simulink model "Con_ref_de_vel"  (R2023b)
settings: Solver=VariableStepAuto  StartTime=0.0  StopTime=14  MaxStep=1e-3  RelTol=1e-3
undefined symbols (not defined in the file or in its folder): alpha_Cu, b_a, b_eq, C_ts, g, J_eq, k_l, K_omega, K_sa, K_sia, K_theta, L_d, L_ls, L_q, lambda_m, magnitude, P_p, r, R_0, R_d, R_q, R_sREF, R_tsamb, T_amb, T_sREF
libraries: simulink x12
(part 1 of 2)
settings Model: Creator=MSI  LastModifiedBy=MSI

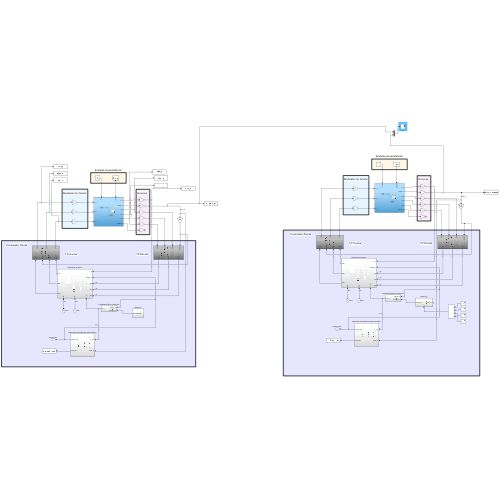
[thumbnail: Simulink's stored preview of the top-level diagram]
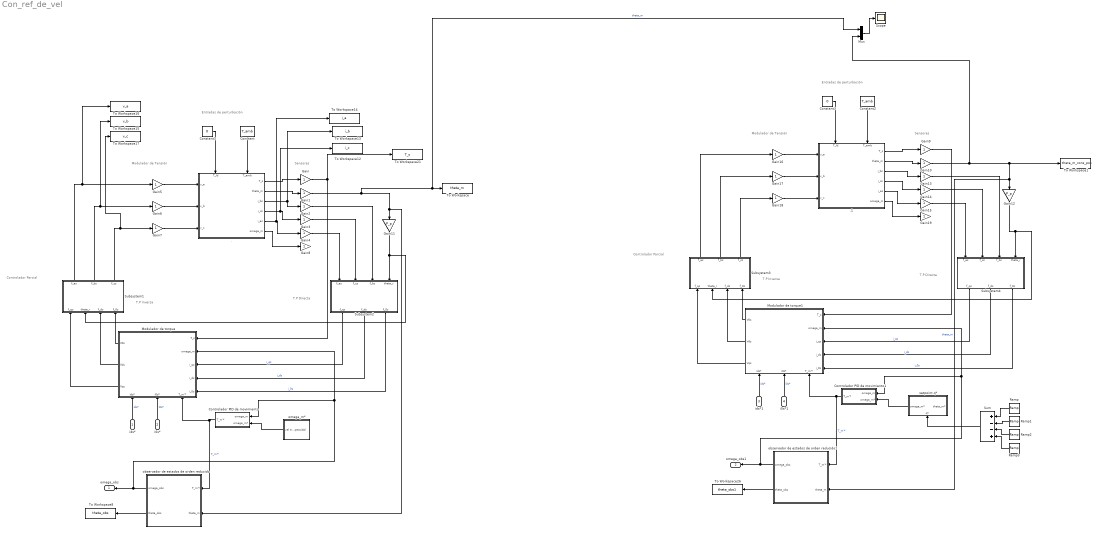
== system Con_ref_de_vel ==
  note: Sensores
  note: T.P Inversa
  note: Entradas de perturbación
  note: Controlador Parcial
  note: T.P Directa
  note: Modulador de Tensión
  note: T.P Directa
  note: Controlador Parcial
  note: Modulador de Tensión
  note: T.P Inversa
  note: Sensores
  note: Entradas de perturbación
  ids* : Inport
  i0s* : Inport  Port=2
  ids*1 : Inport  Port=3
  i0s*1 : Inport  Port=4
  . : Subsystem
      settings: PortSchema="{\"entries\":[{\"content\":{\"sides\":[{\"content\":{\"connectorIds\":[\"In1\",\"In2\",\"In3\"]},\"type\":\"ConnectorPlacement.EquallySpacedRectSide\",\"uuid\":\"a2221977-a2db-4f9f-a6b6-e4e93ab83132\"},{\"content\":{\"connectorIds\":[\"Out1\",\"Out2\",\"Out3\",\"Out4\",\"Out5\",\"Out6\"],\"side\":\"RIGHT\"},\"type\":\"ConnectorPlacement.EquallySpacedRectSide\",\"uuid\":\"4d1b64fb-cd5f-444c-9c55-dd968f667727\"},{\"content\":{\"connectorIds\":[\"In4\",\"In5\"],\"side\":\"TOP\"},\"type\":\"ConnectorPlacement.EquallySpacedRectSide\",\"uuid\":\"feec2d7e-2013-4827-9d2d-5413e6a364ce\"},{\"content\":{\"side\":\"BOTTOM\"},\"type\":\"ConnectorPlacement.EquallySpacedRectSide\",\"uuid\":\"a4e68a75-7272-4a37-88ea-97e0fe693470\"}]},\"type\":\"ConnectorPlacement.EquallySpacedConnector\",\"uuid\":\"3fef7616-1be8-4199-84fe-e5c97ae42ef2\"}],\"packageUris\":[\"http://schema.mathworks.com/mf0/Connector/R2020b\"],\"version\":\"1.0\"}"
  .1 : Subsystem
      settings: PortSchema="{\"entries\":[{\"content\":{\"sides\":[{\"content\":{\"connectorIds\":[\"In1\",\"In2\",\"In3\"]},\"type\":\"ConnectorPlacement.EquallySpacedRectSide\",\"uuid\":\"a2221977-a2db-4f9f-a6b6-e4e93ab83132\"},{\"content\":{\"connectorIds\":[\"Out1\",\"Out2\",\"Out3\",\"Out4\",\"Out5\",\"Out6\"],\"side\":\"RIGHT\"},\"type\":\"ConnectorPlacement.EquallySpacedRectSide\",\"uuid\":\"4d1b64fb-cd5f-444c-9c55-dd968f667727\"},{\"content\":{\"connectorIds\":[\"In4\",\"In5\"],\"side\":\"TOP\"},\"type\":\"ConnectorPlacement.EquallySpacedRectSide\",\"uuid\":\"feec2d7e-2013-4827-9d2d-5413e6a364ce\"},{\"content\":{\"side\":\"BOTTOM\"},\"type\":\"ConnectorPlacement.EquallySpacedRectSide\",\"uuid\":\"a4e68a75-7272-4a37-88ea-97e0fe693470\"}]},\"type\":\"ConnectorPlacement.EquallySpacedConnector\",\"uuid\":\"3fef7616-1be8-4199-84fe-e5c97ae42ef2\"}],\"packageUris\":[\"http://schema.mathworks.com/mf0/Connector/R2020b\"],\"version\":\"1.0\"}"
  Constant : Constant  Value=T_amb
  Constant1 : Constant  Value=0
  Constant2 : Constant  Value=T_amb
  Constant3 : Constant  Value=0
  Controlador PID de movimiento : Subsystem
  Controlador PID de movimiento1 : Subsystem
  Gain{,1..10,13..19} (18 alike) : Gain
  Gain11 : Gain  Gain=P_p
  Gain12 : Gain  Gain=P_p
  Modulador de torque : Subsystem
      settings: PortSchema="{\"entries\":[{\"content\":{\"sides\":[{\"content\":{\"connectorIds\":[\"In1\",\"In2\",\"In3\",\"In4\",\"In5\"]},\"type\":\"ConnectorPlacement.EquallySpacedRectSide\",\"uuid\":\"ba876254-404b-4059-bbdb-b6055672551d\"},{\"content\":{\"connectorIds\":[\"Out1\",\"Out2\",\"Out3\"],\"side\":\"RIGHT\"},\"type\":\"ConnectorPlacement.EquallySpacedRectSide\",\"uuid\":\"d6c00e98-b252-4cfd-8c78-066fe91e4b4f\"},{\"content\":{\"side\":\"TOP\"},\"type\":\"ConnectorPlacement.EquallySpacedRectSide\",\"uuid\":\"a1ad4df6-e3d4-4e16-8862-f0d8c48039a3\"},{\"content\":{\"connectorIds\":[\"In6\",\"In7\",\"In8\"],\"side\":\"BOTTOM\"},\"type\":\"ConnectorPlacement.EquallySpacedRectSide\",\"uuid\":\"e932febf-7e12-4d57-82e2-13690bebd55b\"}]},\"type\":\"ConnectorPlacement.EquallySpacedConnector\",\"uuid\":\"921efeb3-6755-430d-9298-3d05b16ba3fc\"}],\"packageUris\":[\"http://schema.mathworks.com/mf0/Connector/R2020b\"],\"version\":\"1.0\"}"
  Modulador de torque1 : Subsystem
      settings: PortSchema="{\"entries\":[{\"content\":{\"sides\":[{\"content\":{\"connectorIds\":[\"In1\",\"In2\",\"In3\",\"In4\",\"In5\"]},\"type\":\"ConnectorPlacement.EquallySpacedRectSide\",\"uuid\":\"ba876254-404b-4059-bbdb-b6055672551d\"},{\"content\":{\"connectorIds\":[\"Out1\",\"Out2\",\"Out3\"],\"side\":\"RIGHT\"},\"type\":\"ConnectorPlacement.EquallySpacedRectSide\",\"uuid\":\"d6c00e98-b252-4cfd-8c78-066fe91e4b4f\"},{\"content\":{\"side\":\"TOP\"},\"type\":\"ConnectorPlacement.EquallySpacedRectSide\",\"uuid\":\"a1ad4df6-e3d4-4e16-8862-f0d8c48039a3\"},{\"content\":{\"connectorIds\":[\"In6\",\"In7\",\"In8\"],\"side\":\"BOTTOM\"},\"type\":\"ConnectorPlacement.EquallySpacedRectSide\",\"uuid\":\"e932febf-7e12-4d57-82e2-13690bebd55b\"}]},\"type\":\"ConnectorPlacement.EquallySpacedConnector\",\"uuid\":\"921efeb3-6755-430d-9298-3d05b16ba3fc\"}],\"packageUris\":[\"http://schema.mathworks.com/mf0/Connector/R2020b\"],\"version\":\"1.0\"}"
  Mux : Mux  Inputs=2
  Ramp : simulink/Sources/Ramp  slope=(2*pi)/5  start=1  InitialOutput=0
  Ramp1 : simulink/Sources/Ramp  slope=(2*pi)/5  start=6  InitialOutput=0
  Ramp2 : simulink/Sources/Ramp  slope=(2*pi)/5  start=8  InitialOutput=0
  Ramp3 : simulink/Sources/Ramp  slope=(2*pi)/5  start=13  InitialOutput=0
  Scope : Scope
  Subsystem1 : Subsystem
  Subsystem2 : Subsystem
  Subsystem3 : Subsystem
  Subsystem4 : Subsystem
  Sum : Sum  Inputs=+|-|-|+
  To Workspace : ToWorkspace  VariableName=theta_m  SaveFormat=Timeseries  SampleTime=-1
  To Workspace1 : ToWorkspace  VariableName=theta_m_cons_pos  SaveFormat=Timeseries  SampleTime=-1
  To Workspace12 : ToWorkspace  VariableName=i_c  SaveFormat=Timeseries  SampleTime=-1
  To Workspace13 : ToWorkspace  VariableName=i_b  SaveFormat=Timeseries  SampleTime=-1
  To Workspace14 : ToWorkspace  VariableName=i_a  SaveFormat=Timeseries  SampleTime=-1
  To Workspace15 : ToWorkspace  VariableName=v_b  SaveFormat=Timeseries  SampleTime=-1
  To Workspace16 : ToWorkspace  VariableName=v_a  SaveFormat=Timeseries  SampleTime=-1
  To Workspace17 : ToWorkspace  VariableName=v_c  SaveFormat=Timeseries  SampleTime=-1
  To Workspace21 : ToWorkspace  VariableName=T_s  SaveFormat=Timeseries  SampleTime=-1
  To Workspace26 : ToWorkspace  VariableName=theta_obs1  SaveFormat=Timeseries  SampleTime=-1
  To Workspace8 : ToWorkspace  VariableName=theta_obs  SaveFormat=Timeseries  SampleTime=-1
  observador de estados de orden reducido : Subsystem
  observador de estados de orden reducido1 : Subsystem
  omega_m* : Subsystem
  setpoint q* : Subsystem
      settings: PortSchema="{\"entries\":[{\"content\":{\"sides\":[{\"content\":{\"connectorIds\":[\"Out2\"]},\"type\":\"ConnectorPlacement.EquallySpacedRectSide\",\"uuid\":\"9195cc1d-87bf-4a80-b8ff-2f4cc3cb6632\"},{\"content\":{\"connectorIds\":[\"Out1\"],\"side\":\"RIGHT\"},\"type\":\"ConnectorPlacement.EquallySpacedRectSide\",\"uuid\":\"5cc30303-db8f-4b93-aa17-8b0dca3b7a23\"},{\"content\":{\"side\":\"TOP\"},\"type\":\"ConnectorPlacement.EquallySpacedRectSide\",\"uuid\":\"47c6bed7-4bff-4013-bf93-a2b9caf6e24a\"},{\"content\":{\"connectorIds\":[\"In1\"],\"side\":\"BOTTOM\"},\"type\":\"ConnectorPlacement.EquallySpacedRectSide\",\"uuid\":\"27cd8b9a-8a5d-4215-b235-3ab348f130c3\"}]},\"type\":\"ConnectorPlacement.EquallySpacedConnector\",\"uuid\":\"d1d9e87a-f415-4de3-9c74-cafe165ae763\"}],\"packageUris\":[\"http://schema.mathworks.com/mf0/Connector/R2020b\"],\"version\":\"1.0\"}"
  omega_obs : Outport
  omega_obs1 : Outport  Port=2
  wires:
  observador de estados de orden reducido/1(omega_obs) -> omega_obs/1, Modulador de torque/2(omega_m), Controlador PID de movimiento/1(omega_m)
  observador de estados de orden reducido/2(theta_obs) -> To Workspace8/1
  Constant1/1 -> ./4(T_ld)
  Gain2/1 -> Subsystem2/3(f_bs)
  ids*/1 -> Modulador de torque/8(ids*)  "ids*"
  i0s*/1 -> Modulador de torque/7(i0s*)  "i0s*"
  Constant/1 -> ./5(T_amb)
  Subsystem2/2(f_ds) -> Modulador de torque/4(i_ds)  "i_ds"
  Subsystem1/1(f_as) -> To Workspace16/1, Gain5/1
  ./6(omega_m) -> Gain8/1
  Gain11/1 -> Subsystem1/2(theta_r), Subsystem2/4(theta_r)
  Modulador de torque/3(Vqs) -> Subsystem1/1(f_qs)
  Subsystem1/2(f_bs) -> To Workspace15/1, Gain6/1
  Gain7/1 -> ./3(v_c)
  Gain3/1 -> Subsystem2/2(f_cs)
  Subsystem1/3(f_cs) -> To Workspace17/1, Gain7/1
  omega_m*/1(vel trapezoidal) -> Controlador PID de movimiento/2(omega_m*)
  ./3(i_bs) -> To Workspace13/1, Gain2/1
  ./5(i_as) -> To Workspace14/1, Gain4/1
  Controlador PID de movimiento/1(T_m'*) -> observador de estados de orden reducido/1(T_m'*), Modulador de torque/6(T_m'*)  "T_m'*"
  ./2(theta_m) -> Gain1/1
  ./4(i_cs) -> To Workspace12/1, Gain3/1
  Subsystem2/3(f_0s) -> Modulador de torque/5(i_0s)  "i_0s"
  Modulador de torque/1(V0s) -> Subsystem1/4(f_0s)
  Subsystem2/1(f_qs) -> Modulador de torque/3(i_qs)  "i_qs"
  Gain/1 -> Modulador de torque/1(T_s), To Workspace21/1
  Modulador de torque/2(Vds) -> Subsystem1/3(f_ds)
  Gain1/1 -> Mux/1, To Workspace/1, observador de estados de orden reducido/2(theta_m), Gain11/1  "theta_m"
  ./1(T_s) -> Gain/1
  Gain6/1 -> ./2(v_b)
  Gain5/1 -> ./1(v_a)
  Gain4/1 -> Subsystem2/1(f_as)
  Modulador de torque1/3(Vqs) -> Subsystem3/1(f_qs)
  i0s*1/1 -> Modulador de torque1/7(i0s*)  "i0s*"
  Gain10/1 -> Mux/2, To Workspace1/1, observador de estados de orden reducido1/2(theta_m), Gain12/1  "theta_m"
  .1/6(omega_m) -> Gain19/1
  Subsystem3/1(f_as) -> Gain16/1
  .1/3(i_bs) -> Gain13/1
  Gain17/1 -> .1/2(v_b)
  Subsystem4/1(f_qs) -> Modulador de torque1/3(i_qs)  "i_qs"
  .1/2(theta_m) -> Gain10/1
  Modulador de torque1/2(Vds) -> Subsystem3/3(f_ds)
  .1/1(T_s) -> Gain9/1
  Gain18/1 -> .1/3(v_c)
  Subsystem4/2(f_ds) -> Modulador de torque1/4(i_ds)  "i_ds"
  Gain15/1 -> Subsystem4/1(f_as)
  setpoint q*/1(omega_m*) -> Controlador PID de movimiento1/2(omega_m*)
  .1/5(i_as) -> Gain15/1
  Gain9/1 -> Modulador de torque1/1(T_s)
  Subsystem3/2(f_bs) -> Gain17/1
  .1/4(i_cs) -> Gain14/1
  Controlador PID de movimiento1/1(T_m'*) -> observador de estados de orden reducido1/1(T_m'*), Modulador de torque1/6(T_m'*)  "T_m'*"
  Gain14/1 -> Subsystem4/2(f_cs)
  Ramp2/1 -> Sum/3
  Gain13/1 -> Subsystem4/3(f_bs)
  Sum/1 -> setpoint q*/1(q*)
  Ramp/1 -> Sum/1
  ids*1/1 -> Modulador de torque1/8(ids*)  "ids*"
  observador de estados de orden reducido1/2(theta_obs) -> To Workspace26/1
  observador de estados de orden reducido1/1(omega_obs) -> omega_obs1/1, Modulador de torque1/2(omega_m), Controlador PID de movimiento1/1(omega_m)
  Gain12/1 -> Subsystem3/2(theta_r), Subsystem4/4(theta_r)
  Constant3/1 -> .1/4(T_ld)
  Constant2/1 -> .1/5(T_amb)
  Modulador de torque1/1(V0s) -> Subsystem3/4(f_0s)
  Gain16/1 -> .1/1(v_a)
  Ramp1/1 -> Sum/2
  Subsystem4/3(f_0s) -> Modulador de torque1/5(i_0s)  "i_0s"
  Ramp3/1 -> Sum/4
  Subsystem3/3(f_cs) -> Gain18/1
  Mux/1 -> Scope/1

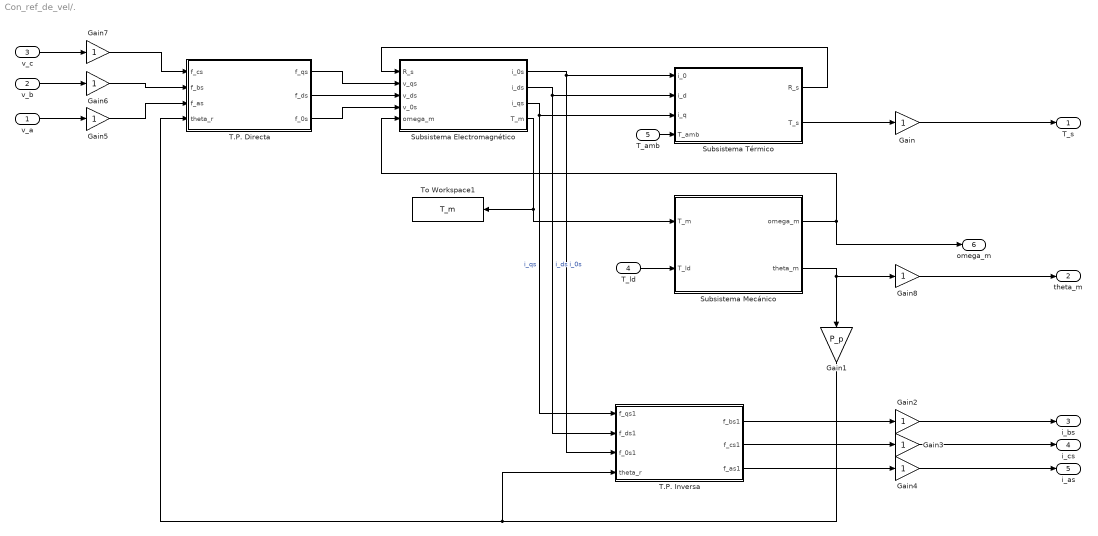
== system Con_ref_de_vel/. ==
  v_a : Inport
  v_b : Inport  Port=2
  v_c : Inport  Port=3
  T_ld : Inport  Port=4
  T_amb : Inport  Port=5
  Gain{,2..8} (8 alike) : Gain
  Gain1 : Gain  Gain=P_p
  Subsistema Electromagnético : Subsystem
  Subsistema Mecánico : Subsystem
  Subsistema Térmico : Subsystem
  T.P. Directa : Subsystem
  T.P. Inversa : Subsystem
  To Workspace1 : ToWorkspace  VariableName=T_m  SaveFormat=Timeseries  SampleTime=-1
  T_s : Outport
  theta_m : Outport  Port=2
  i_bs : Outport  Port=3
  i_cs : Outport  Port=4
  i_as : Outport  Port=5
  omega_m : Outport  Port=6
  wires:
  Subsistema Térmico/1(R_s) -> Subsistema Electromagnético/1(R_s)
  T.P. Directa/1(f_qs) -> Subsistema Electromagnético/2(v_qs)
  T.P. Inversa/1(f_bs1) -> Gain2/1
  Subsistema Mecánico/1(omega_m) -> omega_m/1, Subsistema Electromagnético/5(omega_m)
  Subsistema Electromagnético/1(i_0s) -> Subsistema Térmico/1(i_0), T.P. Inversa/3(f_0s1)  "i_0s"
  Subsistema Mecánico/2(theta_m) -> Gain1/1, Gain8/1
  Gain6/1 -> T.P. Directa/2(f_bs)
  Subsistema Electromagnético/4(T_m) -> Subsistema Mecánico/1(T_m), To Workspace1/1
  Gain3/1 -> i_cs/1
  Subsistema Electromagnético/2(i_ds) -> T.P. Inversa/2(f_ds1), Subsistema Térmico/2(i_d)  "i_ds"
  Gain2/1 -> i_bs/1
  T_amb/1 -> Subsistema Térmico/4(T_amb)
  v_b/1 -> Gain6/1
  v_c/1 -> Gain7/1
  v_a/1 -> Gain5/1
  Subsistema Térmico/2(T_s) -> Gain/1
  Subsistema Electromagnético/3(i_qs) -> T.P. Inversa/1(f_qs1), Subsistema Térmico/3(i_q)  "i_qs"
  Gain4/1 -> i_as/1
  T.P. Inversa/3(f_as1) -> Gain4/1
  T.P. Directa/3(f_0s) -> Subsistema Electromagnético/4(v_0s)
  T_ld/1 -> Subsistema Mecánico/2(T_ld)
  T.P. Inversa/2(f_cs1) -> Gain3/1
  Gain8/1 -> theta_m/1
  Gain7/1 -> T.P. Directa/1(f_cs)
  Gain/1 -> T_s/1
  Gain1/1 -> T.P. Directa/4(theta_r), T.P. Inversa/4(theta_r)
  T.P. Directa/2(f_ds) -> Subsistema Electromagnético/3(v_ds)
  Gain5/1 -> T.P. Directa/3(f_as)

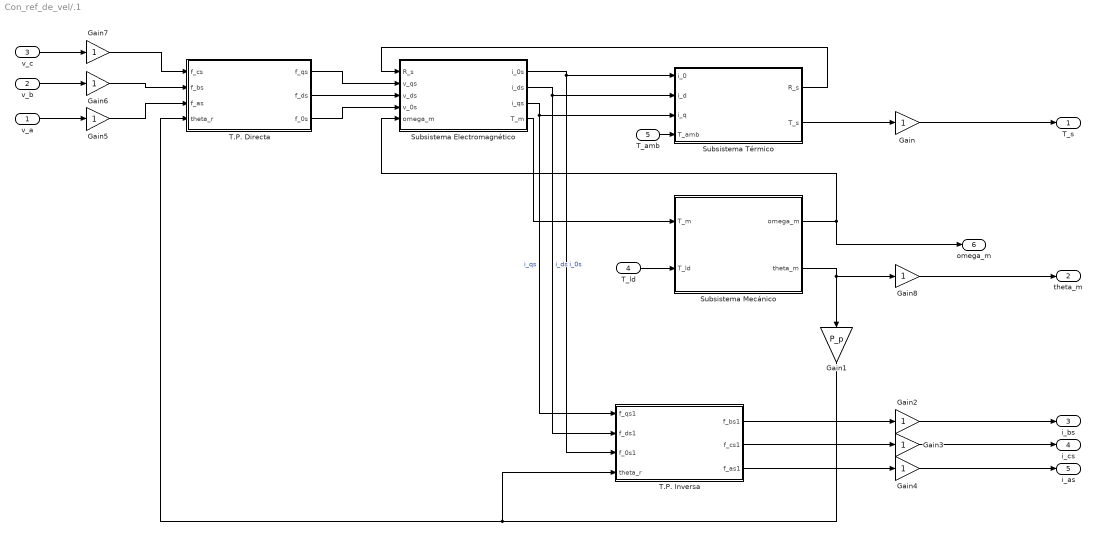
== system Con_ref_de_vel/.1 ==
  v_a : Inport
  v_b : Inport  Port=2
  v_c : Inport  Port=3
  T_ld : Inport  Port=4
  T_amb : Inport  Port=5
  Gain{,2..8} (8 alike) : Gain
  Gain1 : Gain  Gain=P_p
  Subsistema Electromagnético : Subsystem
  Subsistema Mecánico : Subsystem
  Subsistema Térmico : Subsystem
  T.P. Directa : Subsystem
  T.P. Inversa : Subsystem
  T_s : Outport
  theta_m : Outport  Port=2
  i_bs : Outport  Port=3
  i_cs : Outport  Port=4
  i_as : Outport  Port=5
  omega_m : Outport  Port=6
  wires:
  Subsistema Térmico/1(R_s) -> Subsistema Electromagnético/1(R_s)
  T.P. Directa/1(f_qs) -> Subsistema Electromagnético/2(v_qs)
  T.P. Inversa/1(f_bs1) -> Gain2/1
  Subsistema Mecánico/1(omega_m) -> omega_m/1, Subsistema Electromagnético/5(omega_m)
  Subsistema Electromagnético/1(i_0s) -> Subsistema Térmico/1(i_0), T.P. Inversa/3(f_0s1)  "i_0s"
  Subsistema Mecánico/2(theta_m) -> Gain1/1, Gain8/1
  Gain6/1 -> T.P. Directa/2(f_bs)
  Subsistema Electromagnético/4(T_m) -> Subsistema Mecánico/1(T_m)
  Gain3/1 -> i_cs/1
  Subsistema Electromagnético/2(i_ds) -> T.P. Inversa/2(f_ds1), Subsistema Térmico/2(i_d)  "i_ds"
  Gain2/1 -> i_bs/1
  T_amb/1 -> Subsistema Térmico/4(T_amb)
  v_b/1 -> Gain6/1
  v_c/1 -> Gain7/1
  v_a/1 -> Gain5/1
  Subsistema Térmico/2(T_s) -> Gain/1
  Subsistema Electromagnético/3(i_qs) -> T.P. Inversa/1(f_qs1), Subsistema Térmico/3(i_q)  "i_qs"
  Gain4/1 -> i_as/1
  T.P. Inversa/3(f_as1) -> Gain4/1
  T.P. Directa/3(f_0s) -> Subsistema Electromagnético/4(v_0s)
  T_ld/1 -> Subsistema Mecánico/2(T_ld)
  T.P. Inversa/2(f_cs1) -> Gain3/1
  Gain8/1 -> theta_m/1
  Gain7/1 -> T.P. Directa/1(f_cs)
  Gain/1 -> T_s/1
  Gain1/1 -> T.P. Directa/4(theta_r), T.P. Inversa/4(theta_r)
  T.P. Directa/2(f_ds) -> Subsistema Electromagnético/3(v_ds)
  Gain5/1 -> T.P. Directa/3(f_as)

== system Con_ref_de_vel/Controlador PID de movimiento ==
  omega_m : Inport
  omega_m* : Inport  Port=2
  Gain10 : Gain  Gain=K_sa
  Gain12 : Gain  Gain=K_sia
  Gain9 : Gain  Gain=b_a
  Integrator : Integrator
  Integrator1 : Integrator
  Sum : Sum  Inputs=+++
  Sum1 : Sum  Inputs=|-+
  T_m'* : Outport
  wires:
  omega_m*/1 -> Sum1/2
  Integrator/1 -> Integrator1/1, Gain10/1  "e_theta"
  Gain12/1 -> Sum/1
  Integrator1/1 -> Gain12/1
  Sum1/1 -> Gain9/1, Integrator/1  "e_omega_m"
  Sum/1 -> T_m'*/1  "T_m'*"
  Gain9/1 -> Sum/3
  Gain10/1 -> Sum/2
  omega_m/1 -> Sum1/1

== system Con_ref_de_vel/Controlador PID de movimiento1 ==
  omega_m : Inport
  omega_m* : Inport  Port=2
  Gain10 : Gain  Gain=K_sa
  Gain12 : Gain  Gain=K_sia
  Gain9 : Gain  Gain=b_a
  Integrator : Integrator
  Integrator1 : Integrator
  Sum : Sum  Inputs=+++
  Sum1 : Sum  Inputs=|-+
  T_m'* : Outport
  wires:
  omega_m*/1 -> Sum1/2
  Integrator/1 -> Integrator1/1, Gain10/1  "e_theta"
  Gain12/1 -> Sum/1
  Integrator1/1 -> Gain12/1
  Sum1/1 -> Gain9/1, Integrator/1  "e_omega_m"
  Sum/1 -> T_m'*/1  "T_m'*"
  Gain9/1 -> Sum/3
  Gain10/1 -> Sum/2
  omega_m/1 -> Sum1/1

== system Con_ref_de_vel/Modulador de torque ==
  T_s : Inport
  omega_m : Inport  Port=2
  i_qs : Inport  Port=3
  i_ds : Inport  Port=4
  i_0s : Inport  Port=5
  T_m'* : Inport  Port=6
  i0s* : Inport  Port=7
  ids* : Inport  Port=8
  Constant1 : Constant  Value=g
  Desacoplamiento de retroalimentaciones fisicas naturales : Subsystem
      settings: PortSchema="{\"entries\":[{\"content\":{\"sides\":[{\"content\":{\"connectorIds\":[\"In1\",\"In2\",\"In3\",\"In4\",\"In5\"]},\"type\":\"ConnectorPlacement.EquallySpacedRectSide\",\"uuid\":\"229cb02b-d48c-446f-ba32-c62713e9b887\"},{\"content\":{\"connectorIds\":[\"Out1\",\"Out2\",\"Out3\"],\"side\":\"RIGHT\"},\"type\":\"ConnectorPlacement.EquallySpacedRectSide\",\"uuid\":\"d1560b4a-f0ce-405c-b2ec-43a69c5457bd\"},{\"content\":{\"side\":\"TOP\"},\"type\":\"ConnectorPlacement.EquallySpacedRectSide\",\"uuid\":\"c93a9a8d-95cd-44a7-8de3-b4ab0da15153\"},{\"content\":{\"connectorIds\":[\"In6\",\"In7\",\"In8\"],\"side\":\"BOTTOM\"},\"type\":\"ConnectorPlacement.EquallySpacedRectSide\",\"uuid\":\"61b8912b-c246-41e9-a841-420011d131cc\"}]},\"type\":\"ConnectorPlacement.EquallySpacedConnector\",\"uuid\":\"53c75e92-39e8-4743-a399-9153728077fe\"}],\"packageUris\":[\"http://schema.mathworks.com/mf0/Connector/R2020b\"],\"version\":\"1.0\"}"
  Lazo de corriente : Subsystem
      settings: PortSchema="{\"entries\":[{\"content\":{\"sides\":[{\"content\":{\"connectorIds\":[\"In1\",\"In2\",\"In3\",\"In4\"]},\"type\":\"ConnectorPlacement.EquallySpacedRectSide\",\"uuid\":\"e4a1f591-de4c-4bed-9730-a0bdcd595dfe\"},{\"content\":{\"connectorIds\":[\"Out1\",\"Out2\",\"Out3\"],\"side\":\"RIGHT\"},\"type\":\"ConnectorPlacement.EquallySpacedRectSide\",\"uuid\":\"b5219b6b-3019-4355-bcfd-890ee0fb4c54\"},{\"content\":{\"side\":\"TOP\"},\"type\":\"ConnectorPlacement.EquallySpacedRectSide\",\"uuid\":\"3e4154c5-0bb5-4a69-ba55-234c7bde9140\"},{\"content\":{\"connectorIds\":[\"In5\",\"In6\"],\"side\":\"BOTTOM\"},\"type\":\"ConnectorPlacement.EquallySpacedRectSide\",\"uuid\":\"43784307-e678-4ce2-8a7d-2ff65f16c696\"}]},\"type\":\"ConnectorPlacement.EquallySpacedConnector\",\"uuid\":\"60b6d0d3-75d2-4869-ad7d-030d7c987d05\"}],\"packageUris\":[\"http://schema.mathworks.com/mf0/Connector/R2020b\"],\"version\":\"1.0\"}"
  Lazo de torque : Subsystem
  V0s : Outport
  Vds : Outport  Port=2
  Vqs : Outport  Port=3
  wires:
  Lazo de corriente/1(V0s*) -> Desacoplamiento de retroalimentaciones fisicas naturales/6(V0s*)
  ids*/1 -> Lazo de corriente/5(ids*)
  Lazo de corriente/2(Vds*) -> Desacoplamiento de retroalimentaciones fisicas naturales/7(Vds*)
  i0s*/1 -> Lazo de corriente/6(i0s*)
  i_ds/1 -> Desacoplamiento de retroalimentaciones fisicas naturales/4(i_ds), Lazo de corriente/2(i_ds), Lazo de torque/4(i_ds)
  i_0s/1 -> Lazo de corriente/3(i_0s), Desacoplamiento de retroalimentaciones fisicas naturales/5(i_0s)
  omega_m/1 -> Desacoplamiento de retroalimentaciones fisicas naturales/2(omega_m), Lazo de torque/1(omega_m)
  Lazo de corriente/3(Vqs*) -> Desacoplamiento de retroalimentaciones fisicas naturales/8(Vdq*)
  i_qs/1 -> Lazo de corriente/1(i_qs), Desacoplamiento de retroalimentaciones fisicas naturales/3(i_qs)
  Desacoplamiento de retroalimentaciones fisicas naturales/1(Vqs) -> Vqs/1
  Desacoplamiento de retroalimentaciones fisicas naturales/3(V0s) -> V0s/1
  Constant1/1 -> Lazo de torque/3(g)  "g"
  Lazo de torque/1(iqs*) -> Lazo de corriente/4(iqs*)
  T_m'*/1 -> Lazo de torque/2(T_m'*)
  Desacoplamiento de retroalimentaciones fisicas naturales/2(Vds) -> Vds/1
  T_s/1 -> Desacoplamiento de retroalimentaciones fisicas naturales/1(T_s)

== system Con_ref_de_vel/Modulador de torque1 ==
  T_s : Inport
  omega_m : Inport  Port=2
  i_qs : Inport  Port=3
  i_ds : Inport  Port=4
  i_0s : Inport  Port=5
  T_m'* : Inport  Port=6
  i0s* : Inport  Port=7
  ids* : Inport  Port=8
  Constant1 : Constant  Value=g
  Desacoplamiento de retroalimentaciones fisicas naturales : Subsystem
      settings: PortSchema="{\"entries\":[{\"content\":{\"sides\":[{\"content\":{\"connectorIds\":[\"In1\",\"In2\",\"In3\",\"In4\",\"In5\"]},\"type\":\"ConnectorPlacement.EquallySpacedRectSide\",\"uuid\":\"229cb02b-d48c-446f-ba32-c62713e9b887\"},{\"content\":{\"connectorIds\":[\"Out1\",\"Out2\",\"Out3\"],\"side\":\"RIGHT\"},\"type\":\"ConnectorPlacement.EquallySpacedRectSide\",\"uuid\":\"d1560b4a-f0ce-405c-b2ec-43a69c5457bd\"},{\"content\":{\"side\":\"TOP\"},\"type\":\"ConnectorPlacement.EquallySpacedRectSide\",\"uuid\":\"c93a9a8d-95cd-44a7-8de3-b4ab0da15153\"},{\"content\":{\"connectorIds\":[\"In6\",\"In7\",\"In8\"],\"side\":\"BOTTOM\"},\"type\":\"ConnectorPlacement.EquallySpacedRectSide\",\"uuid\":\"61b8912b-c246-41e9-a841-420011d131cc\"}]},\"type\":\"ConnectorPlacement.EquallySpacedConnector\",\"uuid\":\"53c75e92-39e8-4743-a399-9153728077fe\"}],\"packageUris\":[\"http://schema.mathworks.com/mf0/Connector/R2020b\"],\"version\":\"1.0\"}"
  Lazo de corriente : Subsystem
      settings: PortSchema="{\"entries\":[{\"content\":{\"sides\":[{\"content\":{\"connectorIds\":[\"In1\",\"In2\",\"In3\",\"In4\"]},\"type\":\"ConnectorPlacement.EquallySpacedRectSide\",\"uuid\":\"e4a1f591-de4c-4bed-9730-a0bdcd595dfe\"},{\"content\":{\"connectorIds\":[\"Out1\",\"Out2\",\"Out3\"],\"side\":\"RIGHT\"},\"type\":\"ConnectorPlacement.EquallySpacedRectSide\",\"uuid\":\"b5219b6b-3019-4355-bcfd-890ee0fb4c54\"},{\"content\":{\"side\":\"TOP\"},\"type\":\"ConnectorPlacement.EquallySpacedRectSide\",\"uuid\":\"3e4154c5-0bb5-4a69-ba55-234c7bde9140\"},{\"content\":{\"connectorIds\":[\"In5\",\"In6\"],\"side\":\"BOTTOM\"},\"type\":\"ConnectorPlacement.EquallySpacedRectSide\",\"uuid\":\"43784307-e678-4ce2-8a7d-2ff65f16c696\"}]},\"type\":\"ConnectorPlacement.EquallySpacedConnector\",\"uuid\":\"60b6d0d3-75d2-4869-ad7d-030d7c987d05\"}],\"packageUris\":[\"http://schema.mathworks.com/mf0/Connector/R2020b\"],\"version\":\"1.0\"}"
  Lazo de torque : Subsystem
  V0s : Outport
  Vds : Outport  Port=2
  Vqs : Outport  Port=3
  wires:
  Lazo de corriente/1(V0s*) -> Desacoplamiento de retroalimentaciones fisicas naturales/6(V0s*)
  ids*/1 -> Lazo de corriente/5(ids*)
  Lazo de corriente/2(Vds*) -> Desacoplamiento de retroalimentaciones fisicas naturales/7(Vds*)
  i0s*/1 -> Lazo de corriente/6(i0s*)
  i_ds/1 -> Desacoplamiento de retroalimentaciones fisicas naturales/4(i_ds), Lazo de corriente/2(i_ds), Lazo de torque/4(i_ds)
  i_0s/1 -> Lazo de corriente/3(i_0s), Desacoplamiento de retroalimentaciones fisicas naturales/5(i_0s)
  omega_m/1 -> Desacoplamiento de retroalimentaciones fisicas naturales/2(omega_m), Lazo de torque/1(omega_m)
  Lazo de corriente/3(Vqs*) -> Desacoplamiento de retroalimentaciones fisicas naturales/8(Vdq*)
  i_qs/1 -> Lazo de corriente/1(i_qs), Desacoplamiento de retroalimentaciones fisicas naturales/3(i_qs)
  Desacoplamiento de retroalimentaciones fisicas naturales/1(Vqs) -> Vqs/1
  Desacoplamiento de retroalimentaciones fisicas naturales/3(V0s) -> V0s/1
  Constant1/1 -> Lazo de torque/3(g)  "g"
  Lazo de torque/1(iqs*) -> Lazo de corriente/4(iqs*)
  T_m'*/1 -> Lazo de torque/2(T_m'*)
  Desacoplamiento de retroalimentaciones fisicas naturales/2(Vds) -> Vds/1
  T_s/1 -> Desacoplamiento de retroalimentaciones fisicas naturales/1(T_s)

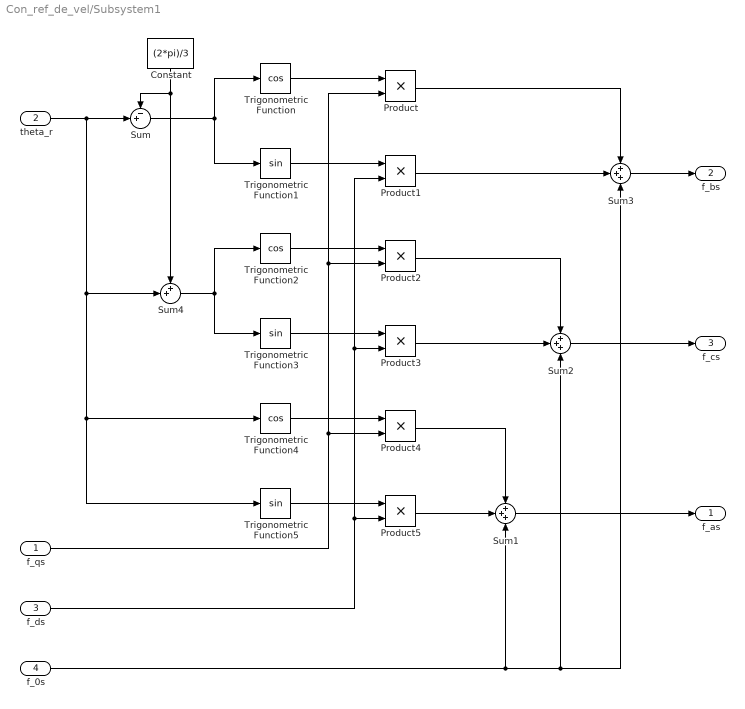
== system Con_ref_de_vel/Subsystem1 ==
  f_qs : Inport
  theta_r : Inport  Port=2
  f_ds : Inport  Port=3
  f_0s : Inport  Port=4
  Constant : Constant  Value=(2*pi)/3
  Product{,1..5} (6 alike) : Product
  Sum : Sum  Inputs=-+|
  Sum1 : Sum  Inputs=+++
  Sum2 : Sum  Inputs=+++
  Sum3 : Sum  Inputs=+++
  Sum4 : Sum  Inputs=++|
  Trigonometric Function : Trigonometry  Operator=cos
  Trigonometric Function1 : Trigonometry
  Trigonometric Function2 : Trigonometry  Operator=cos
  Trigonometric Function3 : Trigonometry
  Trigonometric Function4 : Trigonometry  Operator=cos
  Trigonometric Function5 : Trigonometry
  f_as : Outport
  f_bs : Outport  Port=2
  f_cs : Outport  Port=3
  wires:
  Sum1/1 -> f_as/1
  Product5/1 -> Sum1/2
  Sum2/1 -> f_cs/1
  Product1/1 -> Sum3/2
  Trigonometric Function5/1 -> Product5/1
  Sum/1 -> Trigonometric Function1/1, Trigonometric Function/1
  Product2/1 -> Sum2/1
  Product4/1 -> Sum1/1
  f_qs/1 -> Product4/2, Product2/2, Product/2
  Product/1 -> Sum3/1
  f_0s/1 -> Sum3/3, Sum2/3, Sum1/3
  Trigonometric Function4/1 -> Product4/1
  Constant/1 -> Sum4/1, Sum/1
  Trigonometric Function2/1 -> Product2/1
  f_ds/1 -> Product5/2, Product3/2, Product1/2
  Trigonometric Function3/1 -> Product3/1
  Trigonometric Function1/1 -> Product1/1
  Sum4/1 -> Trigonometric Function3/1, Trigonometric Function2/1
  Sum3/1 -> f_bs/1
  theta_r/1 -> Sum4/2, Trigonometric Function5/1, Trigonometric Function4/1, Sum/2
  Product3/1 -> Sum2/2
  Trigonometric Function/1 -> Product/1

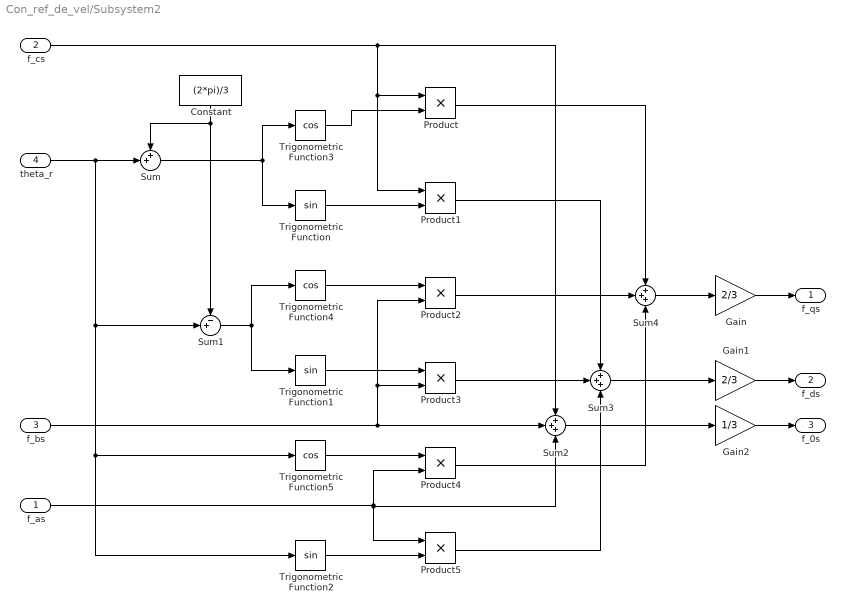
== system Con_ref_de_vel/Subsystem2 ==
  f_as : Inport
  f_cs : Inport  Port=2
  f_bs : Inport  Port=3
  theta_r : Inport  Port=4
  Constant : Constant  Value=(2*pi)/3
  Gain : Gain  Gain=2/3
  Gain1 : Gain  Gain=2/3
  Gain2 : Gain  Gain=1/3
  Product{,1..5} (6 alike) : Product
  Sum : Sum  Inputs=++|
  Sum1 : Sum  Inputs=-+|
  Sum2 : Sum  Inputs=+++
  Sum3 : Sum  Inputs=+++
  Sum4 : Sum  Inputs=+++
  Trigonometric Function : Trigonometry
  Trigonometric Function1 : Trigonometry
  Trigonometric Function2 : Trigonometry
  Trigonometric Function3 : Trigonometry  Operator=cos
  Trigonometric Function4 : Trigonometry  Operator=cos
  Trigonometric Function5 : Trigonometry  Operator=cos
  f_qs : Outport
  f_ds : Outport  Port=2
  f_0s : Outport  Port=3
  wires:
  f_cs/1 -> Product/1, Product1/1, Sum2/1
  Product3/1 -> Sum3/2
  Trigonometric Function5/1 -> Product4/1
  Constant/1 -> Sum/1, Sum1/1
  Sum1/1 -> Trigonometric Function1/1, Trigonometric Function4/1
  Gain2/1 -> f_0s/1
  Gain1/1 -> f_ds/1
  theta_r/1 -> Sum1/2, Trigonometric Function2/1, Trigonometric Function5/1, Sum/2
  Sum4/1 -> Gain/1
  Trigonometric Function1/1 -> Product3/1
  f_bs/1 -> Product2/2, Product3/2, Sum2/2
  Product4/1 -> Sum4/3
  Gain/1 -> f_qs/1
  Product/1 -> Sum4/1
  f_as/1 -> Sum2/3, Product5/1, Product4/2
  Sum2/1 -> Gain2/1
  Product2/1 -> Sum4/2
  Trigonometric Function2/1 -> Product5/2
  Sum3/1 -> Gain1/1
  Trigonometric Function/1 -> Product1/2
  Trigonometric Function3/1 -> Product/2
  Trigonometric Function4/1 -> Product2/1
  Product5/1 -> Sum3/3
  Product1/1 -> Sum3/1
  Sum/1 -> Trigonometric Function3/1, Trigonometric Function/1

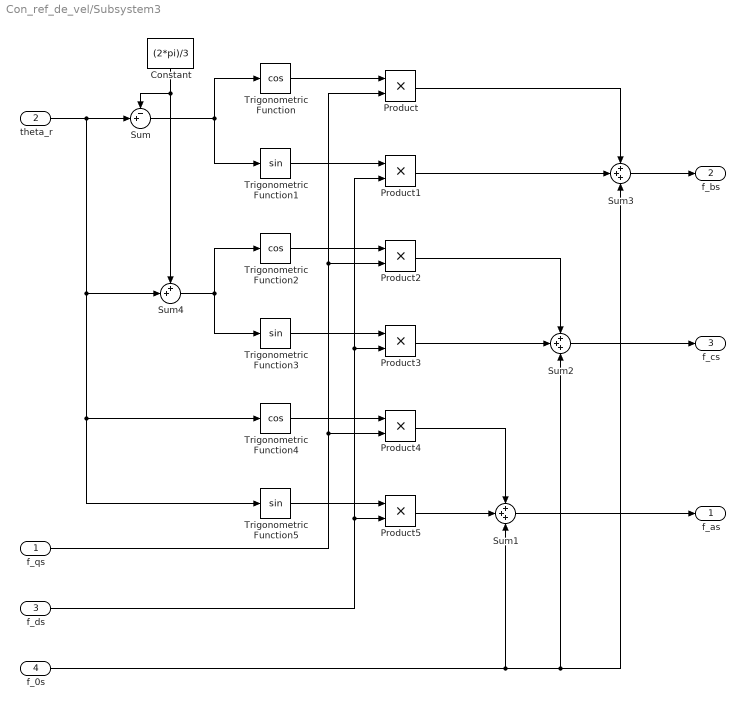
== system Con_ref_de_vel/Subsystem3 ==
  f_qs : Inport
  theta_r : Inport  Port=2
  f_ds : Inport  Port=3
  f_0s : Inport  Port=4
  Constant : Constant  Value=(2*pi)/3
  Product{,1..5} (6 alike) : Product
  Sum : Sum  Inputs=-+|
  Sum1 : Sum  Inputs=+++
  Sum2 : Sum  Inputs=+++
  Sum3 : Sum  Inputs=+++
  Sum4 : Sum  Inputs=++|
  Trigonometric Function : Trigonometry  Operator=cos
  Trigonometric Function1 : Trigonometry
  Trigonometric Function2 : Trigonometry  Operator=cos
  Trigonometric Function3 : Trigonometry
  Trigonometric Function4 : Trigonometry  Operator=cos
  Trigonometric Function5 : Trigonometry
  f_as : Outport
  f_bs : Outport  Port=2
  f_cs : Outport  Port=3
  wires:
  Sum1/1 -> f_as/1
  Product5/1 -> Sum1/2
  Sum2/1 -> f_cs/1
  Product1/1 -> Sum3/2
  Trigonometric Function5/1 -> Product5/1
  Sum/1 -> Trigonometric Function1/1, Trigonometric Function/1
  Product2/1 -> Sum2/1
  Product4/1 -> Sum1/1
  f_qs/1 -> Product4/2, Product2/2, Product/2
  Product/1 -> Sum3/1
  f_0s/1 -> Sum3/3, Sum2/3, Sum1/3
  Trigonometric Function4/1 -> Product4/1
  Constant/1 -> Sum4/1, Sum/1
  Trigonometric Function2/1 -> Product2/1
  f_ds/1 -> Product5/2, Product3/2, Product1/2
  Trigonometric Function3/1 -> Product3/1
  Trigonometric Function1/1 -> Product1/1
  Sum4/1 -> Trigonometric Function3/1, Trigonometric Function2/1
  Sum3/1 -> f_bs/1
  theta_r/1 -> Sum4/2, Trigonometric Function5/1, Trigonometric Function4/1, Sum/2
  Product3/1 -> Sum2/2
  Trigonometric Function/1 -> Product/1

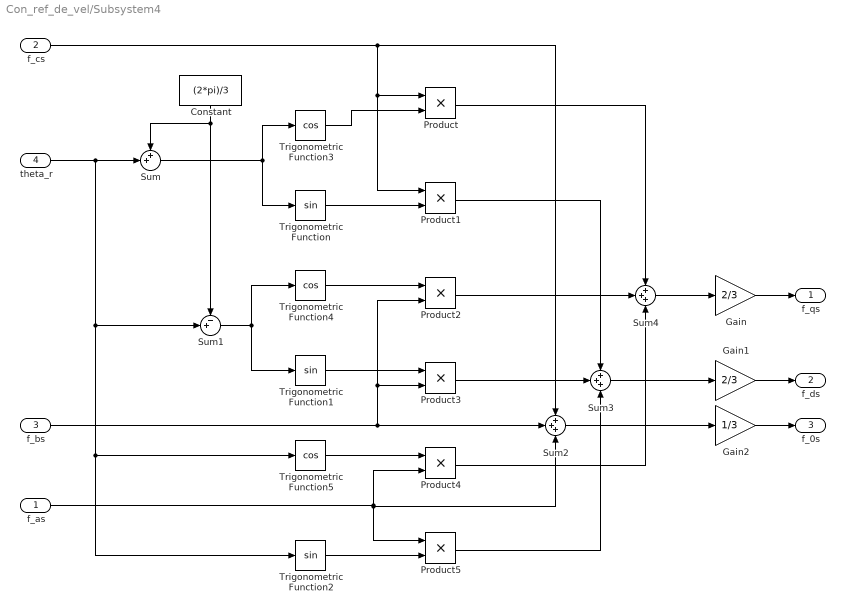
== system Con_ref_de_vel/Subsystem4 ==
  f_as : Inport
  f_cs : Inport  Port=2
  f_bs : Inport  Port=3
  theta_r : Inport  Port=4
  Constant : Constant  Value=(2*pi)/3
  Gain : Gain  Gain=2/3
  Gain1 : Gain  Gain=2/3
  Gain2 : Gain  Gain=1/3
  Product{,1..5} (6 alike) : Product
  Sum : Sum  Inputs=++|
  Sum1 : Sum  Inputs=-+|
  Sum2 : Sum  Inputs=+++
  Sum3 : Sum  Inputs=+++
  Sum4 : Sum  Inputs=+++
  Trigonometric Function : Trigonometry
  Trigonometric Function1 : Trigonometry
  Trigonometric Function2 : Trigonometry
  Trigonometric Function3 : Trigonometry  Operator=cos
  Trigonometric Function4 : Trigonometry  Operator=cos
  Trigonometric Function5 : Trigonometry  Operator=cos
  f_qs : Outport
  f_ds : Outport  Port=2
  f_0s : Outport  Port=3
  wires:
  f_cs/1 -> Product/1, Product1/1, Sum2/1
  Product3/1 -> Sum3/2
  Trigonometric Function5/1 -> Product4/1
  Constant/1 -> Sum/1, Sum1/1
  Sum1/1 -> Trigonometric Function1/1, Trigonometric Function4/1
  Gain2/1 -> f_0s/1
  Gain1/1 -> f_ds/1
  theta_r/1 -> Sum1/2, Trigonometric Function2/1, Trigonometric Function5/1, Sum/2
  Sum4/1 -> Gain/1
  Trigonometric Function1/1 -> Product3/1
  f_bs/1 -> Product2/2, Product3/2, Sum2/2
  Product4/1 -> Sum4/3
  Gain/1 -> f_qs/1
  Product/1 -> Sum4/1
  f_as/1 -> Sum2/3, Product5/1, Product4/2
  Sum2/1 -> Gain2/1
  Product2/1 -> Sum4/2
  Trigonometric Function2/1 -> Product5/2
  Sum3/1 -> Gain1/1
  Trigonometric Function/1 -> Product1/2
  Trigonometric Function3/1 -> Product/2
  Trigonometric Function4/1 -> Product2/1
  Product5/1 -> Sum3/3
  Product1/1 -> Sum3/1
  Sum/1 -> Trigonometric Function3/1, Trigonometric Function/1

== system Con_ref_de_vel/observador de estados de orden reducido ==
  T_m'* : Inport
  theta_m : Inport  Port=2
  Gain10 : Gain  Gain=K_omega
  Gain12 : Gain  Gain=K_theta
  Gain9 : Gain  Gain=1/J_eq
  Integrator : Integrator
  Integrator1 : Integrator
  Sum : Sum  Inputs=++|
  Sum5 : Sum  Inputs=+-
  Sum6 : Sum  Inputs=++|
  omega_obs : Outport
  theta_obs : Outport  Port=2
  wires:
  Sum6/1 -> omega_obs/1, Integrator1/1
  Integrator/1 -> Sum6/2
  Sum5/1 -> Gain10/1, Gain12/1
  T_m'*/1 -> Gain9/1
  Integrator1/1 -> theta_obs/1, Sum5/2
  Gain12/1 -> Sum6/1
  Gain9/1 -> Sum/2
  Gain10/1 -> Sum/1
  theta_m/1 -> Sum5/1
  Sum/1 -> Integrator/1

== system Con_ref_de_vel/observador de estados de orden reducido1 ==
  T_m'* : Inport
  theta_m : Inport  Port=2
  Gain10 : Gain  Gain=K_omega
  Gain12 : Gain  Gain=K_theta
  Gain9 : Gain  Gain=1/J_eq
  Integrator : Integrator
  Integrator1 : Integrator
  Sum : Sum  Inputs=++|
  Sum5 : Sum  Inputs=+-
  Sum6 : Sum  Inputs=++|
  omega_obs : Outport
  theta_obs : Outport  Port=2
  wires:
  Sum6/1 -> omega_obs/1, Integrator1/1
  Integrator/1 -> Sum6/2
  Sum5/1 -> Gain10/1, Gain12/1
  T_m'*/1 -> Gain9/1
  Integrator1/1 -> theta_obs/1, Sum5/2
  Gain12/1 -> Sum6/1
  Gain9/1 -> Sum/2
  Gain10/1 -> Sum/1
  theta_m/1 -> Sum5/1
  Sum/1 -> Integrator/1

== system Con_ref_de_vel/omega_m* ==
  Ramp : simulink/Sources/Ramp  slope=1500  start=1  InitialOutput=0
  Ramp1 : simulink/Sources/Ramp  slope=-1500  start=1.1  InitialOutput=0
  Ramp2 : simulink/Sources/Ramp  slope=-1500  start=5.9  InitialOutput=0
  Ramp3 : simulink/Sources/Ramp  slope=-1500  start=8  InitialOutput=0
  Ramp4 : simulink/Sources/Ramp  slope=1500  start=6  InitialOutput=0
  Ramp5 : simulink/Sources/Ramp  slope=1500  start=8.1  InitialOutput=0
  Ramp6 : simulink/Sources/Ramp  slope=1500  start=12.9  InitialOutput=0
  Ramp7 : simulink/Sources/Ramp  slope=-1500  start=13  InitialOutput=0
  Sum1 : Sum  Inputs=++++++++
  vel trapezoidal : Outport
  wires:
  Ramp4/1 -> Sum1/4
  Ramp2/1 -> Sum1/3
  Ramp3/1 -> Sum1/5
  Ramp1/1 -> Sum1/2
  Ramp6/1 -> Sum1/7
  Ramp/1 -> Sum1/1
  Ramp5/1 -> Sum1/6
  Sum1/1 -> vel trapezoidal/1  "cuadrada"
  Ramp7/1 -> Sum1/8

== system Con_ref_de_vel/setpoint q* ==
  q* : Inport
  Derivative : Derivative
  Gain9 : Gain  Gain=r
  omega_m* : Outport
  theta_m* : Outport  Port=2
  wires:
  Derivative/1 -> omega_m*/1  "omega_m*"
  q*/1 -> Gain9/1
  Gain9/1 -> Derivative/1, theta_m*/1  "theta_m*"

== system Con_ref_de_vel/./Subsistema Electromagnético ==
  R_s : Inport
  v_qs : Inport  Port=2
  v_ds : Inport  Port=3
  v_0s : Inport  Port=4
  omega_m : Inport  Port=5
  corriente_i_0s : Subsystem
  corriente_i_ds : Subsystem
  corriente_i_qs : Subsystem
  torque_T_m : Subsystem
  i_0s : Outport
  i_ds : Outport  Port=2
  i_qs : Outport  Port=3
  T_m : Outport  Port=4
  wires:
  R_s/1 -> corriente_i_qs/3(R_s), corriente_i_ds/4(R_s), corriente_i_0s/2(R_s)
  corriente_i_0s/1(i_0s) -> i_0s/1
  corriente_i_qs/1(i_qs) -> i_qs/1, torque_T_m/2(i_qs), corriente_i_ds/2(i_qs)
  corriente_i_ds/1(i_ds) -> corriente_i_qs/4(i_ds), torque_T_m/1(i_ds), i_ds/1
  v_0s/1 -> corriente_i_0s/1(v_0s)
  v_ds/1 -> corriente_i_ds/1(v_ds)
  omega_m/1 -> corriente_i_qs/1(omega_m), corriente_i_ds/3(omega_m)
  v_qs/1 -> corriente_i_qs/2(v_qs)
  torque_T_m/1(T_m) -> T_m/1

== system Con_ref_de_vel/./Subsistema Mecánico ==
  T_m : Inport
  T_ld : Inport  Port=2
  Constant : Constant  Value=g
  Gain : Gain  Gain=1/J_eq
  Gain1 : Gain  Gain=b_eq
  Gain2 : Gain  Gain=1/r
  Gain3 : Gain  Gain=k_l
  Gain4 : Gain  Gain=1/r
  Product : Product
  Sum : Sum  Inputs=-+-
  Sum1 : Sum
  Trigonometric Function : Trigonometry
  "omega_m(0) = 0\t" : Integrator
  theta_m(0) = 0 : Integrator
  omega_m : Outport
  theta_m : Outport  Port=2
  wires:
  Product/1 -> Sum1/2
  Constant/1 -> Product/1
  T_m/1 -> Sum/2
  Gain3/1 -> Product/2
  T_ld/1 -> Sum1/1
  Gain1/1 -> Sum/3
  Gain4/1 -> Sum/1
  Sum1/1 -> Gain4/1  "T_l"
  theta_m(0) = 0/1 -> Gain2/1, theta_m/1  "theta_m(t)"
  Trigonometric Function/1 -> Gain3/1
  Sum/1 -> Gain/1
  Gain2/1 -> Trigonometric Function/1
  "omega_m(0) = 0\t"/1 -> theta_m(0) = 0/1, omega_m/1, Gain1/1  "omega_m(t)"
  Gain/1 -> "omega_m(0) = 0\t"/1  "domega_m(t)/dt"

== system Con_ref_de_vel/./Subsistema Térmico ==
  i_0 : Inport
  i_d : Inport  Port=2
  i_q : Inport  Port=3
  T_amb : Inport  Port=4
  Constant : Constant
  Constant1 : Constant  Value=T_sREF
  Gain : Gain  Gain=R_sREF
  Gain1 : Gain  Gain=alpha_Cu
  Gain5 : Gain  Gain=2
  Gain6 : Gain  Gain=3/2
  Gain7 : Gain  Gain=1/R_tsamb
  Gain8 : Gain  Gain=1/C_ts
  Math Function1 : Math  Operator=magnitude^2  OutputSignalType=real
  Math Function2 : Math  Operator=magnitude^2  OutputSignalType=real
  Math Function3 : Math  Operator=magnitude^2  OutputSignalType=real
  Product1 : Product
  Sum : Sum  Inputs=|++
  Sum1 : Sum  Inputs=|+-
  Sum2 : Sum  Inputs=+|+|+
  Sum3 : Sum  Inputs=-+|
  Sum4 : Sum  Inputs=-+|
  T_s(0) = T_amb : Integrator  InitialCondition=T_amb
  R_s : Outport
  T_s : Outport  Port=2
  wires:
  i_q/1 -> Math Function2/1
  i_d/1 -> Math Function3/1
  i_0/1 -> Math Function1/1
  Gain1/1 -> Sum/1
  Gain8/1 -> T_s(0) = T_amb/1
  Sum3/1 -> Gain8/1
  Constant/1 -> Sum/2
  Product1/1 -> Sum3/2
  Sum/1 -> Gain/1
  T_amb/1 -> Sum4/1
  Math Function1/1 -> Gain5/1
  Sum4/1 -> Gain7/1
  T_s(0) = T_amb/1 -> Sum1/1, Sum4/2, T_s/1
  Sum2/1 -> Gain6/1
  Sum1/1 -> Gain1/1
  Gain6/1 -> Product1/1
  Constant1/1 -> Sum1/2
  Gain5/1 -> Sum2/3
  Gain7/1 -> Sum3/1
  Math Function2/1 -> Sum2/1
  Math Function3/1 -> Sum2/2
  Gain/1 -> R_s/1, Product1/2

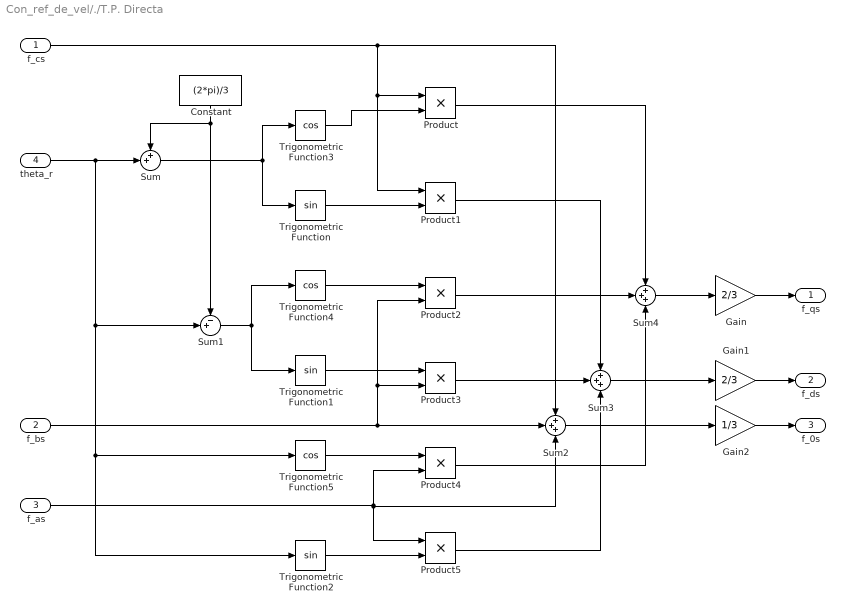
== system Con_ref_de_vel/./T.P. Directa ==
  f_cs : Inport
  f_bs : Inport  Port=2
  f_as : Inport  Port=3
  theta_r : Inport  Port=4
  Constant : Constant  Value=(2*pi)/3
  Gain : Gain  Gain=2/3
  Gain1 : Gain  Gain=2/3
  Gain2 : Gain  Gain=1/3
  Product{,1..5} (6 alike) : Product
  Sum : Sum  Inputs=++|
  Sum1 : Sum  Inputs=-+|
  Sum2 : Sum  Inputs=+++
  Sum3 : Sum  Inputs=+++
  Sum4 : Sum  Inputs=+++
  Trigonometric Function : Trigonometry
  Trigonometric Function1 : Trigonometry
  Trigonometric Function2 : Trigonometry
  Trigonometric Function3 : Trigonometry  Operator=cos
  Trigonometric Function4 : Trigonometry  Operator=cos
  Trigonometric Function5 : Trigonometry  Operator=cos
  f_qs : Outport
  f_ds : Outport  Port=2
  f_0s : Outport  Port=3
  wires:
  Product5/1 -> Sum3/3
  theta_r/1 -> Sum1/2, Trigonometric Function2/1, Trigonometric Function5/1, Sum/2
  f_bs/1 -> Product2/2, Product3/2, Sum2/2
  f_cs/1 -> Product/1, Product1/1, Sum2/1
  Trigonometric Function5/1 -> Product4/1
  Sum1/1 -> Trigonometric Function1/1, Trigonometric Function4/1
  Constant/1 -> Sum/1, Sum1/1
  Sum/1 -> Trigonometric Function3/1, Trigonometric Function/1
  f_as/1 -> Sum2/3, Product5/1, Product4/2
  Gain2/1 -> f_0s/1
  Trigonometric Function2/1 -> Product5/2
  Trigonometric Function1/1 -> Product3/1
  Product/1 -> Sum4/1
  Sum4/1 -> Gain/1
  Trigonometric Function3/1 -> Product/2
  Gain/1 -> f_qs/1
  Gain1/1 -> f_ds/1
  Product2/1 -> Sum4/2
  Product1/1 -> Sum3/1
  Product4/1 -> Sum4/3
  Product3/1 -> Sum3/2
  Sum2/1 -> Gain2/1
  Trigonometric Function4/1 -> Product2/1
  Trigonometric Function/1 -> Product1/2
  Sum3/1 -> Gain1/1

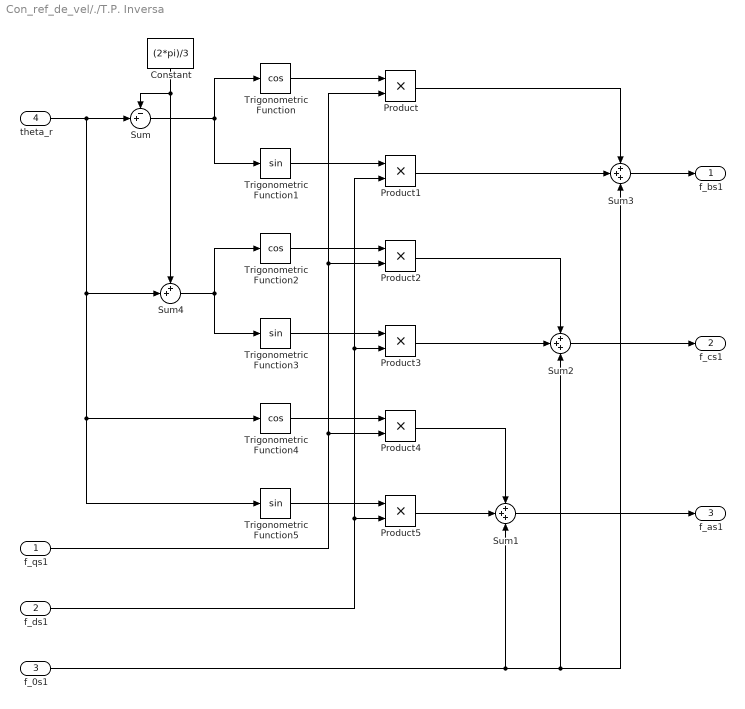
== system Con_ref_de_vel/./T.P. Inversa ==
  f_qs1 : Inport
  f_ds1 : Inport  Port=2
  f_0s1 : Inport  Port=3
  theta_r : Inport  Port=4
  Constant : Constant  Value=(2*pi)/3
  Product{,1..5} (6 alike) : Product
  Sum : Sum  Inputs=-+|
  Sum1 : Sum  Inputs=+++
  Sum2 : Sum  Inputs=+++
  Sum3 : Sum  Inputs=+++
  Sum4 : Sum  Inputs=++|
  Trigonometric Function : Trigonometry  Operator=cos
  Trigonometric Function1 : Trigonometry
  Trigonometric Function2 : Trigonometry  Operator=cos
  Trigonometric Function3 : Trigonometry
  Trigonometric Function4 : Trigonometry  Operator=cos
  Trigonometric Function5 : Trigonometry
  f_bs1 : Outport
  f_cs1 : Outport  Port=2
  f_as1 : Outport  Port=3
  wires:
  theta_r/1 -> Sum4/2, Trigonometric Function5/1, Trigonometric Function4/1, Sum/2
  Trigonometric Function3/1 -> Product3/1
  Product4/1 -> Sum1/1
  Product1/1 -> Sum3/2
  Trigonometric Function2/1 -> Product2/1
  Product2/1 -> Sum2/1
  f_0s1/1 -> Sum3/3, Sum2/3, Sum1/3
  f_qs1/1 -> Product4/2, Product2/2, Product/2
  Product5/1 -> Sum1/2
  Trigonometric Function1/1 -> Product1/1
  Sum/1 -> Trigonometric Function1/1, Trigonometric Function/1
  Trigonometric Function5/1 -> Product5/1
  Sum4/1 -> Trigonometric Function3/1, Trigonometric Function2/1
  Product/1 -> Sum3/1
  Product3/1 -> Sum2/2
  Trigonometric Function/1 -> Product/1
  Sum2/1 -> f_cs1/1
  Sum3/1 -> f_bs1/1
  f_ds1/1 -> Product5/2, Product3/2, Product1/2
  Trigonometric Function4/1 -> Product4/1
  Sum1/1 -> f_as1/1
  Constant/1 -> Sum4/1, Sum/1

== system Con_ref_de_vel/.1/Subsistema Electromagnético ==
  R_s : Inport
  v_qs : Inport  Port=2
  v_ds : Inport  Port=3
  v_0s : Inport  Port=4
  omega_m : Inport  Port=5
  corriente_i_0s : Subsystem
  corriente_i_ds : Subsystem
  corriente_i_qs : Subsystem
  torque_T_m : Subsystem
  i_0s : Outport
  i_ds : Outport  Port=2
  i_qs : Outport  Port=3
  T_m : Outport  Port=4
  wires:
  R_s/1 -> corriente_i_qs/3(R_s), corriente_i_ds/4(R_s), corriente_i_0s/2(R_s)
  corriente_i_0s/1(i_0s) -> i_0s/1
  corriente_i_qs/1(i_qs) -> i_qs/1, torque_T_m/2(i_qs), corriente_i_ds/2(i_qs)
  corriente_i_ds/1(i_ds) -> corriente_i_qs/4(i_ds), torque_T_m/1(i_ds), i_ds/1
  v_0s/1 -> corriente_i_0s/1(v_0s)
  v_ds/1 -> corriente_i_ds/1(v_ds)
  omega_m/1 -> corriente_i_qs/1(omega_m), corriente_i_ds/3(omega_m)
  v_qs/1 -> corriente_i_qs/2(v_qs)
  torque_T_m/1(T_m) -> T_m/1

== system Con_ref_de_vel/.1/Subsistema Mecánico ==
  T_m : Inport
  T_ld : Inport  Port=2
  Constant : Constant  Value=g
  Gain : Gain  Gain=1/J_eq
  Gain1 : Gain  Gain=b_eq
  Gain2 : Gain  Gain=1/r
  Gain3 : Gain  Gain=k_l
  Gain4 : Gain  Gain=1/r
  Product : Product
  Sum : Sum  Inputs=-+-
  Sum1 : Sum
  Trigonometric Function : Trigonometry
  "omega_m(0) = 0\t" : Integrator
  theta_m(0) = 0 : Integrator
  omega_m : Outport
  theta_m : Outport  Port=2
  wires:
  Product/1 -> Sum1/2
  Constant/1 -> Product/1
  T_m/1 -> Sum/2
  Gain3/1 -> Product/2
  T_ld/1 -> Sum1/1
  Gain1/1 -> Sum/3
  Gain4/1 -> Sum/1
  Sum1/1 -> Gain4/1  "T_l"
  theta_m(0) = 0/1 -> Gain2/1, theta_m/1  "theta_m(t)"
  Trigonometric Function/1 -> Gain3/1
  Sum/1 -> Gain/1
  Gain2/1 -> Trigonometric Function/1
  "omega_m(0) = 0\t"/1 -> theta_m(0) = 0/1, omega_m/1, Gain1/1  "omega_m(t)"
  Gain/1 -> "omega_m(0) = 0\t"/1  "domega_m(t)/dt"

== system Con_ref_de_vel/.1/Subsistema Térmico ==
  i_0 : Inport
  i_d : Inport  Port=2
  i_q : Inport  Port=3
  T_amb : Inport  Port=4
  Constant : Constant
  Constant1 : Constant  Value=T_sREF
  Gain : Gain  Gain=R_sREF
  Gain1 : Gain  Gain=alpha_Cu
  Gain5 : Gain  Gain=2
  Gain6 : Gain  Gain=3/2
  Gain7 : Gain  Gain=1/R_tsamb
  Gain8 : Gain  Gain=1/C_ts
  Math Function1 : Math  Operator=magnitude^2  OutputSignalType=real
  Math Function2 : Math  Operator=magnitude^2  OutputSignalType=real
  Math Function3 : Math  Operator=magnitude^2  OutputSignalType=real
  Product1 : Product
  Sum : Sum  Inputs=|++
  Sum1 : Sum  Inputs=|+-
  Sum2 : Sum  Inputs=+|+|+
  Sum3 : Sum  Inputs=-+|
  Sum4 : Sum  Inputs=-+|
  T_s(0) = T_amb : Integrator  InitialCondition=T_amb
  R_s : Outport
  T_s : Outport  Port=2
  wires:
  i_q/1 -> Math Function2/1
  i_d/1 -> Math Function3/1
  i_0/1 -> Math Function1/1
  Gain1/1 -> Sum/1
  Gain8/1 -> T_s(0) = T_amb/1
  Sum3/1 -> Gain8/1
  Constant/1 -> Sum/2
  Product1/1 -> Sum3/2
  Sum/1 -> Gain/1
  T_amb/1 -> Sum4/1
  Math Function1/1 -> Gain5/1
  Sum4/1 -> Gain7/1
  T_s(0) = T_amb/1 -> Sum1/1, Sum4/2, T_s/1
  Sum2/1 -> Gain6/1
  Sum1/1 -> Gain1/1
  Gain6/1 -> Product1/1
  Constant1/1 -> Sum1/2
  Gain5/1 -> Sum2/3
  Gain7/1 -> Sum3/1
  Math Function2/1 -> Sum2/1
  Math Function3/1 -> Sum2/2
  Gain/1 -> R_s/1, Product1/2

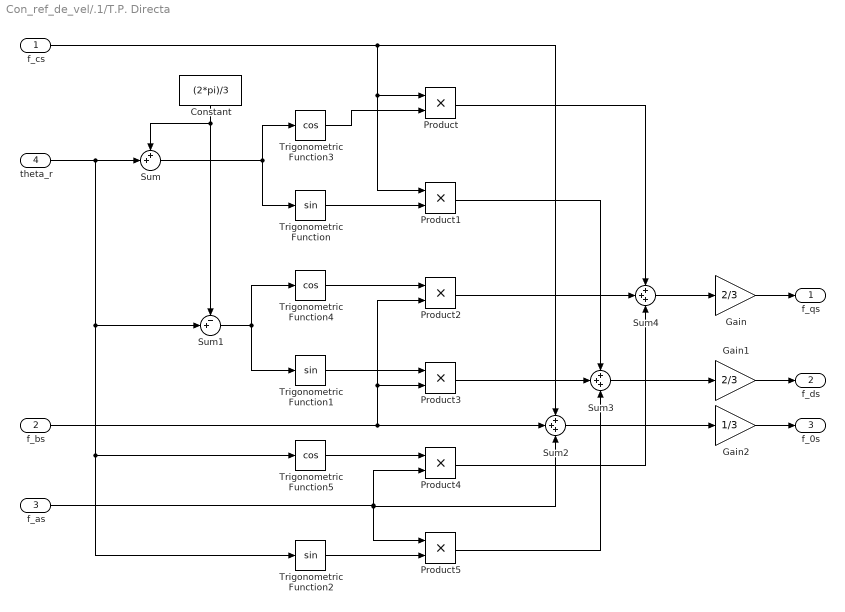
== system Con_ref_de_vel/.1/T.P. Directa ==
  f_cs : Inport
  f_bs : Inport  Port=2
  f_as : Inport  Port=3
  theta_r : Inport  Port=4
  Constant : Constant  Value=(2*pi)/3
  Gain : Gain  Gain=2/3
  Gain1 : Gain  Gain=2/3
  Gain2 : Gain  Gain=1/3
  Product{,1..5} (6 alike) : Product
  Sum : Sum  Inputs=++|
  Sum1 : Sum  Inputs=-+|
  Sum2 : Sum  Inputs=+++
  Sum3 : Sum  Inputs=+++
  Sum4 : Sum  Inputs=+++
  Trigonometric Function : Trigonometry
  Trigonometric Function1 : Trigonometry
  Trigonometric Function2 : Trigonometry
  Trigonometric Function3 : Trigonometry  Operator=cos
  Trigonometric Function4 : Trigonometry  Operator=cos
  Trigonometric Function5 : Trigonometry  Operator=cos
  f_qs : Outport
  f_ds : Outport  Port=2
  f_0s : Outport  Port=3
  wires:
  Product5/1 -> Sum3/3
  theta_r/1 -> Sum1/2, Trigonometric Function2/1, Trigonometric Function5/1, Sum/2
  f_bs/1 -> Product2/2, Product3/2, Sum2/2
  f_cs/1 -> Product/1, Product1/1, Sum2/1
  Trigonometric Function5/1 -> Product4/1
  Sum1/1 -> Trigonometric Function1/1, Trigonometric Function4/1
  Constant/1 -> Sum/1, Sum1/1
  Sum/1 -> Trigonometric Function3/1, Trigonometric Function/1
  f_as/1 -> Sum2/3, Product5/1, Product4/2
  Gain2/1 -> f_0s/1
  Trigonometric Function2/1 -> Product5/2
  Trigonometric Function1/1 -> Product3/1
  Product/1 -> Sum4/1
  Sum4/1 -> Gain/1
  Trigonometric Function3/1 -> Product/2
  Gain/1 -> f_qs/1
  Gain1/1 -> f_ds/1
  Product2/1 -> Sum4/2
  Product1/1 -> Sum3/1
  Product4/1 -> Sum4/3
  Product3/1 -> Sum3/2
  Sum2/1 -> Gain2/1
  Trigonometric Function4/1 -> Product2/1
  Trigonometric Function/1 -> Product1/2
  Sum3/1 -> Gain1/1

== system Con_ref_de_vel/.1/T.P. Inversa ==
  f_qs1 : Inport
  f_ds1 : Inport  Port=2
  f_0s1 : Inport  Port=3
  theta_r : Inport  Port=4
  Constant : Constant  Value=(2*pi)/3
  Product{,1..5} (6 alike) : Product
  Sum : Sum  Inputs=-+|
  Sum1 : Sum  Inputs=+++
  Sum2 : Sum  Inputs=+++
  Sum3 : Sum  Inputs=+++
  Sum4 : Sum  Inputs=++|
  Trigonometric Function : Trigonometry  Operator=cos
  Trigonometric Function1 : Trigonometry
  Trigonometric Function2 : Trigonometry  Operator=cos
  Trigonometric Function3 : Trigonometry
  Trigonometric Function4 : Trigonometry  Operator=cos
  Trigonometric Function5 : Trigonometry
  f_bs1 : Outport
  f_cs1 : Outport  Port=2
  f_as1 : Outport  Port=3
  wires:
  theta_r/1 -> Sum4/2, Trigonometric Function5/1, Trigonometric Function4/1, Sum/2
  Trigonometric Function3/1 -> Product3/1
  Product4/1 -> Sum1/1
  Product1/1 -> Sum3/2
  Trigonometric Function2/1 -> Product2/1
  Product2/1 -> Sum2/1
  f_0s1/1 -> Sum3/3, Sum2/3, Sum1/3
  f_qs1/1 -> Product4/2, Product2/2, Product/2
  Product5/1 -> Sum1/2
  Trigonometric Function1/1 -> Product1/1
  Sum/1 -> Trigonometric Function1/1, Trigonometric Function/1
  Trigonometric Function5/1 -> Product5/1
  Sum4/1 -> Trigonometric Function3/1, Trigonometric Function2/1
  Product/1 -> Sum3/1
  Product3/1 -> Sum2/2
  Trigonometric Function/1 -> Product/1
  Sum2/1 -> f_cs1/1
  Sum3/1 -> f_bs1/1
  f_ds1/1 -> Product5/2, Product3/2, Product1/2
  Trigonometric Function4/1 -> Product4/1
  Sum1/1 -> f_as1/1
  Constant/1 -> Sum4/1, Sum/1

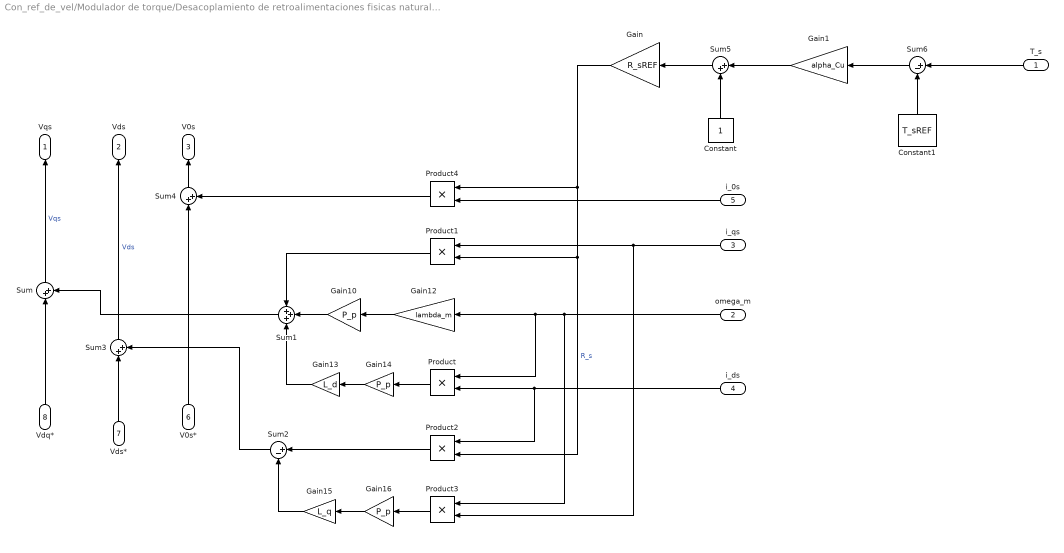
== system Con_ref_de_vel/Modulador de torque/Desacoplamiento de retroalimentaciones fisicas naturales ==
  T_s : Inport
  omega_m : Inport  Port=2
  i_qs : Inport  Port=3
  i_ds : Inport  Port=4
  i_0s : Inport  Port=5
  V0s* : Inport  Port=6
  Vds* : Inport  Port=7
  Vdq* : Inport  Port=8
  Constant : Constant
  Constant1 : Constant  Value=T_sREF
  Gain : Gain  Gain=R_sREF
  Gain1 : Gain  Gain=alpha_Cu
  Gain10 : Gain  Gain=P_p
  Gain12 : Gain  Gain=lambda_m
  Gain13 : Gain  Gain=L_d
  Gain14 : Gain  Gain=P_p
  Gain15 : Gain  Gain=L_q
  Gain16 : Gain  Gain=P_p
  Product{,1..4} (5 alike) : Product
  Sum{,3..5} (4 alike) : Sum  Inputs=|++
  Sum1 : Sum  Inputs=+++
  Sum2 : Sum  Inputs=|+-
  Sum6 : Sum  Inputs=|+-
  Vqs : Outport
  Vds : Outport  Port=2
  V0s : Outport  Port=3
  wires:
  Gain10/1 -> Sum1/2
  Gain13/1 -> Sum1/3
  Gain12/1 -> Gain10/1
  i_qs/1 -> Product3/2, Product1/1
  i_ds/1 -> Product2/1, Product/2
  Gain16/1 -> Gain15/1
  Product2/1 -> Sum2/1
  Product3/1 -> Gain16/1
  Gain/1 -> Product2/2, Product1/2, Product4/1  "R_s"
  Gain15/1 -> Sum2/2
  Product1/1 -> Sum1/1
  Sum2/1 -> Sum3/2
  Sum1/1 -> Sum/2
  Product/1 -> Gain14/1
  omega_m/1 -> Product3/1, Product/1, Gain12/1
  Gain14/1 -> Gain13/1
  Sum3/1 -> Vds/1  "Vds"
  Sum/1 -> Vqs/1  "Vqs"
  i_0s/1 -> Product4/2
  Product4/1 -> Sum4/2
  Sum4/1 -> V0s/1
  Constant1/1 -> Sum6/2
  T_s/1 -> Sum6/1
  Constant/1 -> Sum5/2
  Sum5/1 -> Gain/1
  Sum6/1 -> Gain1/1
  Gain1/1 -> Sum5/1
  Vdq*/1 -> Sum/1
  Vds*/1 -> Sum3/1
  V0s*/1 -> Sum4/1

== system Con_ref_de_vel/Modulador de torque/Lazo de corriente ==
  i_qs : Inport
  i_ds : Inport  Port=2
  i_0s : Inport  Port=3
  iqs* : Inport  Port=4
  ids* : Inport  Port=5
  i0s* : Inport  Port=6
  Gain10 : Gain  Gain=R_d
  Gain12 : Gain  Gain=R_0
  Gain9 : Gain  Gain=R_q
  Sum : Sum  Inputs=|-+
  Sum1 : Sum  Inputs=|-+
  Sum2 : Sum  Inputs=|-+
  V0s* : Outport
  Vds* : Outport  Port=2
  Vqs* : Outport  Port=3
  wires:
  Gain9/1 -> Vqs*/1  "Vqs*"
  Sum/1 -> Gain9/1
  Gain10/1 -> Vds*/1  "Vds*"
  i_qs/1 -> Sum/1
  ids*/1 -> Sum1/2
  i_0s/1 -> Sum2/1
  Sum2/1 -> Gain12/1
  Sum1/1 -> Gain10/1
  i0s*/1 -> Sum2/2
  iqs*/1 -> Sum/2
  i_ds/1 -> Sum1/1
  Gain12/1 -> V0s*/1  "V0s*"

== system Con_ref_de_vel/Modulador de torque/Lazo de torque ==
  omega_m : Inport
  T_m'* : Inport  Port=2
  g : Inport  Port=3
  i_ds : Inport  Port=4
  Constant4 : Constant  Value=L_d
  Constant5 : Constant  Value=L_q
  Constant6 : Constant  Value=lambda_m
  Divide1 : Product  Inputs=*/
  Gain16 : Gain  Gain=b_eq
  Gain17 : Gain  Gain=1/r
  Gain18 : Gain  Gain=k_l
  Gain19 : Gain  Gain=1/r
  Gain20 : Gain  Gain=P_p
  Gain21 : Gain  Gain=3/2
  Integrator1 : Integrator
  Product1 : Product
  Product3 : Product
  Sin1 : Trigonometry
  Sum3 : Sum  Inputs=+++
  Sum4 : Sum  Inputs=-+
  Sum5 : Sum  Inputs=|++
  iqs* : Outport
  wires:
  Integrator1/1 -> Gain17/1
  Product1/1 -> Sum3/3
  Constant6/1 -> Sum5/2
  Gain16/1 -> Sum3/2
  T_m'*/1 -> Sum3/1
  Gain21/1 -> Divide1/2
  g/1 -> Product1/2
  Constant5/1 -> Sum4/1
  Product3/1 -> Sum5/1
  Sum5/1 -> Gain20/1
  Gain18/1 -> Gain19/1
  Sum3/1 -> Divide1/1
  Divide1/1 -> iqs*/1  "iqs*"
  Gain20/1 -> Gain21/1
  Sum4/1 -> Product3/2
  Gain19/1 -> Product1/1
  Gain17/1 -> Sin1/1
  omega_m/1 -> Gain16/1, Integrator1/1
  Sin1/1 -> Gain18/1
  i_ds/1 -> Product3/1
  Constant4/1 -> Sum4/2

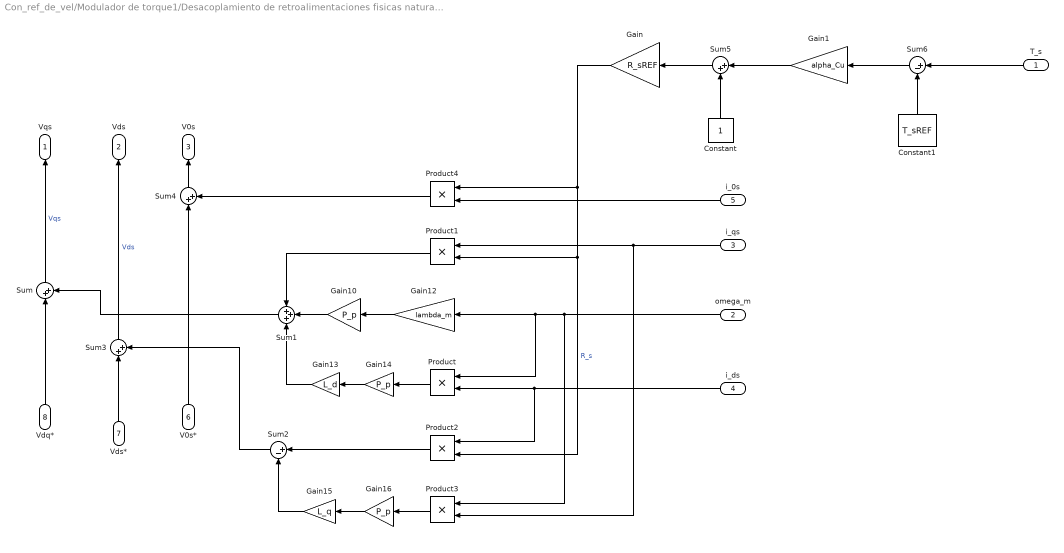
== system Con_ref_de_vel/Modulador de torque1/Desacoplamiento de retroalimentaciones fisicas naturales ==
  T_s : Inport
  omega_m : Inport  Port=2
  i_qs : Inport  Port=3
  i_ds : Inport  Port=4
  i_0s : Inport  Port=5
  V0s* : Inport  Port=6
  Vds* : Inport  Port=7
  Vdq* : Inport  Port=8
  Constant : Constant
  Constant1 : Constant  Value=T_sREF
  Gain : Gain  Gain=R_sREF
  Gain1 : Gain  Gain=alpha_Cu
  Gain10 : Gain  Gain=P_p
  Gain12 : Gain  Gain=lambda_m
  Gain13 : Gain  Gain=L_d
  Gain14 : Gain  Gain=P_p
  Gain15 : Gain  Gain=L_q
  Gain16 : Gain  Gain=P_p
  Product{,1..4} (5 alike) : Product
  Sum{,3..5} (4 alike) : Sum  Inputs=|++
  Sum1 : Sum  Inputs=+++
  Sum2 : Sum  Inputs=|+-
  Sum6 : Sum  Inputs=|+-
  Vqs : Outport
  Vds : Outport  Port=2
  V0s : Outport  Port=3
  wires:
  Gain10/1 -> Sum1/2
  Gain13/1 -> Sum1/3
  Gain12/1 -> Gain10/1
  i_qs/1 -> Product3/2, Product1/1
  i_ds/1 -> Product2/1, Product/2
  Gain16/1 -> Gain15/1
  Product2/1 -> Sum2/1
  Product3/1 -> Gain16/1
  Gain/1 -> Product2/2, Product1/2, Product4/1  "R_s"
  Gain15/1 -> Sum2/2
  Product1/1 -> Sum1/1
  Sum2/1 -> Sum3/2
  Sum1/1 -> Sum/2
  Product/1 -> Gain14/1
  omega_m/1 -> Product3/1, Product/1, Gain12/1
  Gain14/1 -> Gain13/1
  Sum3/1 -> Vds/1  "Vds"
  Sum/1 -> Vqs/1  "Vqs"
  i_0s/1 -> Product4/2
  Product4/1 -> Sum4/2
  Sum4/1 -> V0s/1
  Constant1/1 -> Sum6/2
  T_s/1 -> Sum6/1
  Constant/1 -> Sum5/2
  Sum5/1 -> Gain/1
  Sum6/1 -> Gain1/1
  Gain1/1 -> Sum5/1
  Vdq*/1 -> Sum/1
  Vds*/1 -> Sum3/1
  V0s*/1 -> Sum4/1

== system Con_ref_de_vel/Modulador de torque1/Lazo de corriente ==
  i_qs : Inport
  i_ds : Inport  Port=2
  i_0s : Inport  Port=3
  iqs* : Inport  Port=4
  ids* : Inport  Port=5
  i0s* : Inport  Port=6
  Gain10 : Gain  Gain=R_d
  Gain12 : Gain  Gain=R_0
  Gain9 : Gain  Gain=R_q
  Sum : Sum  Inputs=|-+
  Sum1 : Sum  Inputs=|-+
  Sum2 : Sum  Inputs=|-+
  V0s* : Outport
  Vds* : Outport  Port=2
  Vqs* : Outport  Port=3
  wires:
  Gain9/1 -> Vqs*/1  "Vqs*"
  Sum/1 -> Gain9/1
  Gain10/1 -> Vds*/1  "Vds*"
  i_qs/1 -> Sum/1
  ids*/1 -> Sum1/2
  i_0s/1 -> Sum2/1
  Sum2/1 -> Gain12/1
  Sum1/1 -> Gain10/1
  i0s*/1 -> Sum2/2
  iqs*/1 -> Sum/2
  i_ds/1 -> Sum1/1
  Gain12/1 -> V0s*/1  "V0s*"
